simulink model "power_steppermotor"  (R2015b)
settings: Solver=FixedStepDiscrete  StartTime=0.0  StopTime=0.12  FixedStep=Ts  MaxStep=2e-6
PreLoadFcn:
  | assignin('base','Ts',0.5*1e-8);
InitFcn:
  | Ts=0.5*1e-8;
undefined symbols (not defined in the file): DiscIntNeverNeededParam, sigbuilder_block
libraries: powerlib x7
Description:
  | Copyright 2008-2015 The MathWorks, Inc.
settings Model: ExtModeAutoUpdateStatusClock=off  Creator=MathWorks  LastModifiedBy=YogurtSuee
settings DataIOCC: SaveFormat=Array  SignalLoggingSaveFormat=ModelDataLogs
settings OptimizationCC: ExpressionDepthLimit=2147483647  InitFltsAndDblsToZero=on
settings DebuggingCC: UnderspecifiedInitializationDetection=Classic  MergeDetectMultiDrivingBlocksExec=none  SignalResolutionControl=TryResolveAllWithWarning  SolverPrmCheckMsg=warning  FcnCallInpInsideContextMsg=UseLocalSettings  StateNameClashWarn=warning
settings HardwareCC: ProdBitPerPointer=32  ProdLargestAtomicFloat=None  ProdIntDivRoundTo=Undefined  ProdEndianess=Unspecified  ProdWordSize=32  ProdHWDeviceType=32-bit Generic
settings GRTTargetCC: GeneratePreprocessorConditionals=Disable all  CombineOutputUpdateFcns=off  GRTInterface=on
settings ConfigComp: CovModelRefEnable=Off  CovSFcnEnable=off

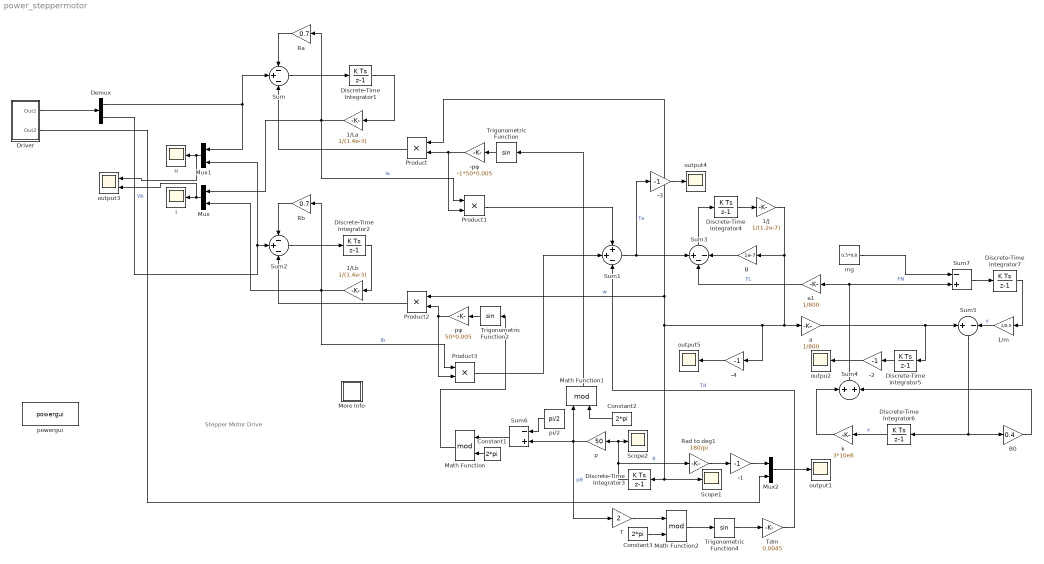
== system power_steppermotor ==
  note: Stepper Motor Drive
  -{1..4} (4 alike) : Gain  Gain=-1
  -pφ : Gain  Gain=-1*50*0.005
  1/J : Gain  Gain=1/(1.2e-7)
  1/La : Gain  Gain=1/(1.4e-3)
  1/Lb : Gain  Gain=1/(1.4e-3)
  1/m : Gain  Gain=1/0.5
  B : Gain  Gain=1e-7
  B0 : Gain  Gain=0.4
  Constant1 : Constant  Value=2*pi
  Constant2 : Constant  Value=2*pi
  Constant3 : Constant  Value=2*pi
  Demux : Demux  Outputs=2
  Discrete-Time Integrator{1..7} (7 alike) : DiscreteIntegrator  SampleTime=Ts  ICPrevOutput=DiscIntNeverNeededParam  ICPrevScaledInput=DiscIntNeverNeededParam
  Driver : Subsystem
  Math Function : Math  Operator=mod  SaturateOnIntegerOverflow=on
  Math Function1 : Math  Operator=mod  SaturateOnIntegerOverflow=on
  Math Function2 : Math  Operator=mod  SaturateOnIntegerOverflow=on
  More Info : Subsystem
      settings: OpenFcn=showdemo(bdroot(gcb))
      mask Display: disp('?')
  Mux : Mux  Inputs=2
  Mux1 : Mux  Inputs=2
  Mux2 : Mux  Inputs=2
  Product{,1..3} (4 alike) : Product
  Ra : Gain  Gain=0.7
  Rad to deg1 : Gain  Gain=180/pi
  Rb : Gain  Gain=0.7
  Scope1 : Scope
  Scope2 : Scope
  Sum : Sum  Inputs=-+-
  Sum1 : Sum  Inputs=++-
  Sum2 : Sum  Inputs=-+-
  Sum3 : Sum  Inputs=+--
  Sum4 : Sum
  Sum5 : Sum  Inputs=+-
  Sum6 : Sum  Inputs=-+
  Sum7 : Sum  Inputs=-+
  T : Gain  Gain=2
  Tdm : Gain  Gain=0.0045
  Trigonometric Function : Trigonometry
  Trigonometric Function2 : Trigonometry
  Trigonometric Function4 : Trigonometry
  a : Gain  Gain=1/800
  a1 : Gain  Gain=1/800
  i : Scope
  k : Gain  Gain=3*10e8
  mg : Constant  Value=0.5*9.8
  outpu2 : Scope
  output1 : Scope
  output3 : Scope  NumInputPorts=2
  output4 : Scope
  output5 : Scope
  p : Gain  Gain=50
  pi/2 : Constant  Value=pi/2
  powergui : powerlib/powergui  SimulationMode=Discrete  SolverType=Tustin/Backward Euler (TBE)  SampleTime=Ts  frequency=60  SPID=off  DisableSnubberDevices=off  DisableRonSwitches=off  DisableVfSwitches=off  SwTol=0  DisplayEquations=off  Interpol=off  ExternalGateDelay=off  methode=off  Ts=0  FunctionMessages=off  echomessages=off  HookPort=off  EnableUseOfTLC=off  x0status=blocks  frequencyindice=0  Pbase=100e6  ErrMax=1e-4  Iterations=50  UnitsV=V  UnitsW=W  buscounter=0  RestoreLinks=warning  ResistiveCurrentMeasurement=off  Frange=[0:2:500]  Ylog=off  Xlog=on  ShowGrid=off  save=off  variable=ZData  structure=0  ZoomFFT=on  StartTime=0.0  cycles=1  DisplayStyle=1  fundamental=60  FreqAxis=off  MaxFrequency=1000  frequencyindicesteady=1  RmsSteady=1  display=off
  pφ : Gain  Gain=50*0.005
  u : Scope
  wires:
  Discrete-Time Integrator1/1 -> 1/La/1
  Sum/1 -> Discrete-Time Integrator1/1
  Ra/1 -> Sum/1
  1/La/1 -> Product1/1, Mux/1, Ra/1  "Ia"
  Product/1 -> Sum/3
  -pφ/1 -> Product/2, Product1/2
  Product1/1 -> Sum1/1
  Discrete-Time Integrator2/1 -> 1/Lb/1
  Sum2/1 -> Discrete-Time Integrator2/1
  Rb/1 -> Sum2/1
  1/Lb/1 -> Product3/1, Mux/2, Rb/1  "Ib"
  Product2/1 -> Sum2/3
  pφ/1 -> Product2/2, Product3/2
  Product3/1 -> Sum1/2
  Tdm/1 -> Sum1/3  "Td"
  1/J/1 -> -4/1, Product2/1, Product/1, Discrete-Time Integrator3/1, Scope1/1, a/1, B/1  "w"
  Sum3/1 -> Discrete-Time Integrator4/1
  Discrete-Time Integrator4/1 -> 1/J/1
  Discrete-Time Integrator3/1 -> Rad to deg1/1, Scope2/1, p/1  "θ"
  p/1 -> Sum6/2, T/1, Math Function1/1  "pθ"
  pi/2/1 -> Sum6/1
  Mux/1 -> output3/2, i/1
  Mux1/1 -> output3/1, u/1
  Trigonometric Function4/1 -> Tdm/1
  Constant1/1 -> Math Function/2
  Sum6/1 -> Math Function/1
  Math Function/1 -> Trigonometric Function2/1
  Constant2/1 -> Math Function1/2
  Math Function1/1 -> Trigonometric Function/1
  Constant3/1 -> Math Function2/2
  T/1 -> Math Function2/1
  Math Function2/1 -> Trigonometric Function4/1
  Sum1/1 -> -3/1, Sum3/1  "Te"
  B/1 -> Sum3/3
  Trigonometric Function/1 -> -pφ/1
  Trigonometric Function2/1 -> pφ/1
  Demux/2 -> Mux1/2, Sum2/2  "Vb"
  Demux/1 -> Mux1/1, Sum/2
  Rad to deg1/1 -> -1/1
  Sum4/1 -> Sum7/2, a1/1  "FN"
  a/1 -> Discrete-Time Integrator5/1, Sum5/1
  mg/1 -> Sum7/1
  Sum7/1 -> Discrete-Time Integrator7/1
  Discrete-Time Integrator7/1 -> 1/m/1
  1/m/1 -> Sum5/2  "v"
  a1/1 -> Sum3/2  "TL"
  Sum5/1 -> Discrete-Time Integrator6/1, B0/1
  Discrete-Time Integrator6/1 -> k/1  "x"
  k/1 -> Sum4/1
  B0/1 -> Sum4/2
  Discrete-Time Integrator5/1 -> -2/1
  Driver/1(Out1) -> Demux/1
  Driver/2(Out2) -> Mux2/2
  Mux2/1 -> output1/1
  -1/1 -> Mux2/1
  -2/1 -> outpu2/1
  -3/1 -> output4/1
  -4/1 -> output5/1

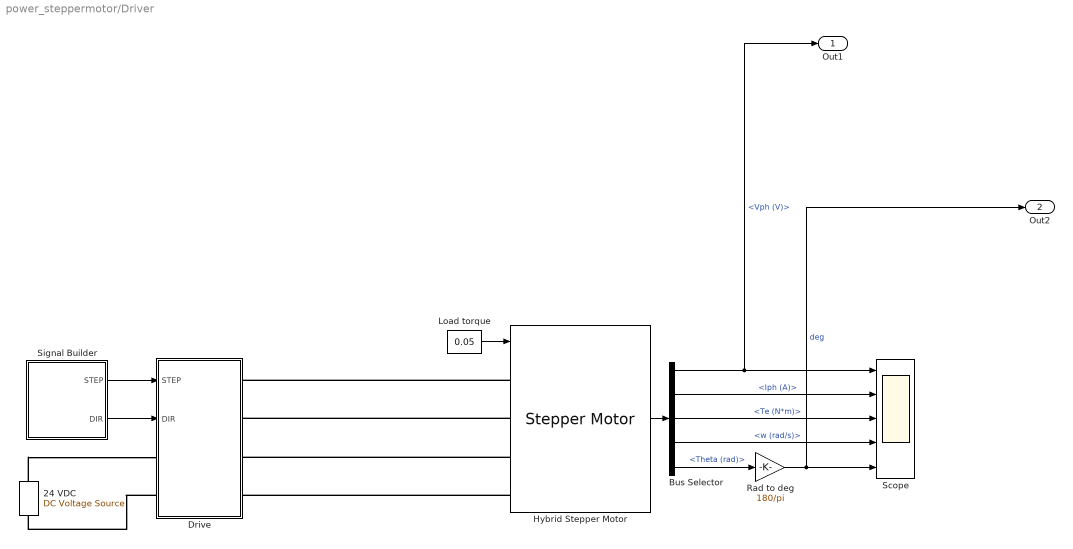
== system power_steppermotor/Driver ==
  24 VDC : powerlib/Electrical Sources/DC Voltage Source  Amplitude=24  Measurements=None
  Bus Selector : BusSelector  OutputSignals=Vph (V),Iph (A),Te (N*m),w (rad/s),Theta (rad)
  Drive : Subsystem  mask{Iref=2, step=200, Ts=Ts}
      mask prompts: Iref "Phase current (A)"; step "Stepping rate (step/s)"; Ts "Sampling time (s)"
      mask init:
      | Nstep=round(1/step/Ts);
  Hybrid Stepper Motor : powerlib/Machines/Stepper Motor  MotorType=Permanent-magnet / Hybrid  NumberOfPhases_1=2  NumberOfPhases_2=3  PresetModel_1=<empty>  PresetModel_2=<empty>  L=1.4e-3  Lmax=10e-3  Lmin=2e-3  R=0.7  Step_angle=1.8  Psim=0.005  Tdm=0.002  J=1.2e-7  B=1e-7*1000  w0=0  pos0=0  TsPowergui=0  TsBlock=-1
  Load torque : Constant  Value=0.05
  Rad to deg : Gain  Gain=180/pi
  Scope : Scope  NumInputPorts=5
  Signal Builder : Subsystem  Tag=STV Subsys  LoadFcn=sigbuilder_block('load');  StartFcn=sigbuilder_block('start');  StopFcn=sigbuilder_block('stop');  ClipboardFcn=sigbuilder_block('clipboard');  mask(Sigbuilder block){}
      mask help: Sigbuilder GUI
      mask init:
      | if ~strcmp(get_param(bdroot(gcbh),'SimulationStatus'),'stopped') tuvar = sigbuilder_block('maskInit'); end
      settings: CopyFcn=sigbuilder_block('copy');  DeleteFcn=sigbuilder_block('delete');  ModelCloseFcn=sigbuilder_block('modelClose');  PreSaveFcn=sigbuilder_block('preSave');  PauseFcn=sigbuilder_block('pause')  ContinueFcn=sigbuilder_block('continue')  NameChangeFcn=sigbuilder_block('namechange');  OpenFcn=sigbuilder_block('open',[162.75 86.25 550.5 363.75 ]);  CloseFcn=sigbuilder_block('close');
      mask Display: plot(0,0,100,100,[10,10,40,40,10],[80,20,20,80,80],[40,10],[50,50], [40,27,10],[65,72,56],[40,25,25,10],[28,28,43,43]);
  Out1 : Outport
  Out2 : Outport  Port=2
  wires:
  Signal Builder/1(STEP) -> Drive/1(STEP)
  Signal Builder/2(DIR) -> Drive/2(DIR)
  Hybrid Stepper Motor/1 -> Bus Selector/1
  Bus Selector/5 -> Rad to deg/1  "<Theta (rad)>"
  Bus Selector/4 -> Scope/4  "<w (rad/s)>"
  Bus Selector/3 -> Scope/3  "<Te (N*m)>"
  Bus Selector/2 -> Scope/2  "<Iph (A)>"
  Load torque/1 -> Hybrid Stepper Motor/1
  Bus Selector/1 -> Out1/1, Scope/1  "<Vph (V)>"
  Rad to deg/1 -> Out2/1, Scope/5  "deg"
  connections:
  24 VDC/RConn1 -- Drive/LConn1
  Hybrid Stepper Motor/LConn4 -- Drive/RConn4
  Hybrid Stepper Motor/LConn1 -- Drive/RConn1
  Drive/LConn2 -- 24 VDC/LConn1
  Hybrid Stepper Motor/LConn3 -- Drive/RConn3
  Hybrid Stepper Motor/LConn2 -- Drive/RConn2

== system power_steppermotor/More Info ==

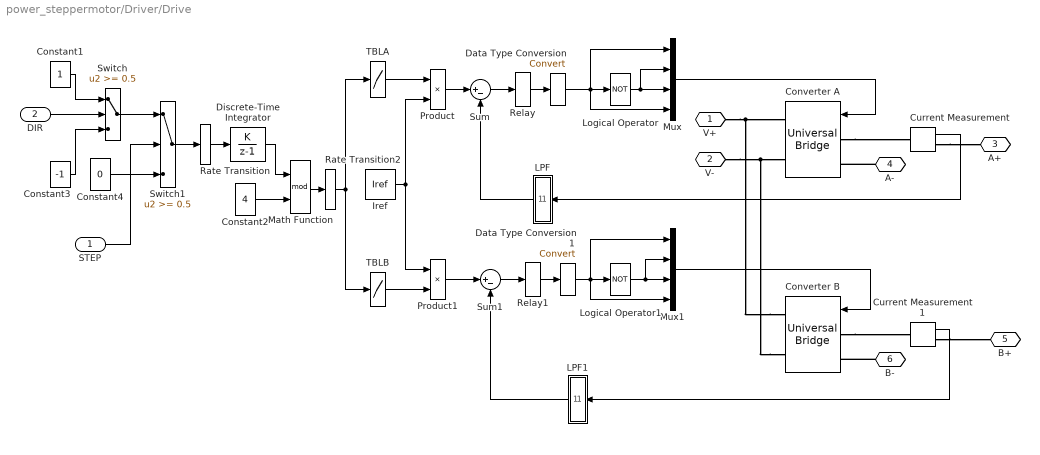
== system power_steppermotor/Driver/Drive ==
  STEP : Inport
  DIR : Inport  Port=2
  Constant1 : Constant  SampleTime=Ts
  Constant2 : Constant  Value=4  SampleTime=Nstep*Ts
  Constant3 : Constant  Value=-1  SampleTime=Ts
  Constant4 : Constant  Value=0  SampleTime=Ts
  Converter A : powerlib/Power Electronics/Universal Bridge  Arms=2  SnubberResistance=10000  SnubberCapacitance=inf  Device=MOSFET / Diodes  Ron=1e-3*10  Lon=0  ForwardVoltages="[  0  0  ]"  ForwardVoltage=0  GTOparameters=[ 10e-6 , 20e-6 ]  IGBTparameters=[ 0.5e-6 , 0.5e-6 ]  Measurements=None  Measurements_2=None  converterType=Rectifier
  Converter B : powerlib/Power Electronics/Universal Bridge  Arms=2  SnubberResistance=10000  SnubberCapacitance=inf  Device=MOSFET / Diodes  Ron=1e-3*10  Lon=0  ForwardVoltages="[  0  0  ]"  ForwardVoltage=0  GTOparameters=[ 10e-6 , 20e-6 ]  IGBTparameters=[ 0.5e-6 , 0.5e-6 ]  Measurements=None  Measurements_2=None  converterType=Rectifier
  Current Measurement : powerlib/Measurements/Current Measurement  PhasorSimulation=off  OutputType=Complex  PSBequivalent=0
  Current Measurement1 : powerlib/Measurements/Current Measurement  PhasorSimulation=off  OutputType=Complex  PSBequivalent=0
  Data Type Conversion : DataTypeConversion
  Data Type Conversion1 : DataTypeConversion
  Discrete-Time Integrator : DiscreteIntegrator  IntegratorMethod=Accumulation: Forward Euler  SampleTime=Nstep*Ts  ICPrevOutput=DiscIntNeverNeededParam  ICPrevScaledInput=DiscIntNeverNeededParam
  Iref : Constant  Value=Iref  SampleTime=Ts
  LPF : Subsystem  mask{fc=10000, Ts=Ts}
      mask prompts: fc "Cut-off frequency (Hz)"; Ts "Sampling time (s)"
      mask init:
      | % fa=tf(1,[1/2/pi/fc 1]);
      | % fn=c2d(fa,Ts);
      | % [NN,DD]=tfdata(fn,'v')
      | 
      | NN = [ 0,0.0609];
      | DD = [1.0000,-0.9391];
  LPF1 : Subsystem  mask{fc=10000, Ts=Ts}
      mask prompts: fc "Cut-off frequency (Hz)"; Ts "Sampling time (s)"
      mask init:
      | % fa=tf(1,[1/2/pi/fc 1]);
      | % fn=c2d(fa,Ts);
      | % [NN,DD]=tfdata(fn,'v')
      | 
      | NN = [ 0,0.0609];
      | DD = [1.0000,-0.9391];
  Logical Operator : Logic  Operator=NOT  AllPortsSameDT=off  OutDataTypeStr=boolean
  Logical Operator1 : Logic  Operator=NOT  AllPortsSameDT=off  OutDataTypeStr=boolean
  Math Function : Math  Operator=mod  SampleTime=Nstep*Ts  SaturateOnIntegerOverflow=on
  Mux : Mux
  Mux1 : Mux
  Product : Product  RndMeth=Zero
  Product1 : Product  RndMeth=Zero
  Rate Transition : RateTransition
  Rate Transition2 : RateTransition
  Relay : Relay  OnSwitchValue=0.01  OffSwitchValue=-0.01
  Relay1 : Relay  OnSwitchValue=0.01  OffSwitchValue=-0.01  OutDataTypeStr=Inherit: Inherit via back propagation
  Sum : Sum  Inputs=|+-  OutDataTypeStr=Inherit: Same as first input
  Sum1 : Sum  Inputs=|+-  OutDataTypeStr=Inherit: Same as first input
  Switch : Switch  Threshold=0.5  ZeroCross=off  SampleTime=Ts
  Switch1 : Switch  Threshold=0.5  ZeroCross=off  SampleTime=Ts
  TBLA : Lookup  InputValues=[0:3]  Table=[1 0 -1 0]  SampleTime=Ts
  TBLB : Lookup  InputValues=[0:3]  Table=[0 1 0 -1]  SampleTime=Ts
  V+ : PMIOPort  Port=1  Side=Left
  V- : PMIOPort  Port=2  Side=Left
  A+ : PMIOPort  Port=3  Side=Right
  A- : PMIOPort  Port=4  Side=Right
  B+ : PMIOPort  Port=5  Side=Right
  B- : PMIOPort  Port=6  Side=Right
  wires:
  Constant4/1 -> Switch1/3
  Switch1/1 -> Rate Transition/1
  Switch/1 -> Switch1/1
  STEP/1 -> Switch1/2
  DIR/1 -> Switch/2
  Rate Transition2/1 -> TBLB/1, TBLA/1
  Math Function/1 -> Rate Transition2/1
  Product1/1 -> Sum1/1
  Product/1 -> Sum/1
  Rate Transition/1 -> Discrete-Time Integrator/1
  Constant3/1 -> Switch/3
  Constant1/1 -> Switch/1
  Discrete-Time Integrator/1 -> Math Function/1
  Constant2/1 -> Math Function/2
  Iref/1 -> Product1/1, Product/2
  TBLB/1 -> Product1/2
  TBLA/1 -> Product/1
  LPF1/1(O) -> Sum1/2
  LPF/1(O) -> Sum/2
  Data Type Conversion1/1 -> Mux1/4, Mux1/1, Logical Operator1/1
  Data Type Conversion/1 -> Logical Operator/1, Mux/4, Mux/1
  Current Measurement1/1 -> LPF1/1(I)
  Sum1/1 -> Relay1/1
  Mux1/1 -> Converter B/1
  Logical Operator1/1 -> Mux1/2, Mux1/3
  Relay1/1 -> Data Type Conversion1/1
  Mux/1 -> Converter A/1
  Logical Operator/1 -> Mux/2, Mux/3
  Relay/1 -> Data Type Conversion/1
  Current Measurement/1 -> LPF/1(I)
  Sum/1 -> Relay/1
  connections:
  Converter B/RConn2 -- Converter A/RConn2 -- V-/RConn1
  Converter B/RConn1 -- Converter A/RConn1 -- V+/RConn1
  Current Measurement1/RConn1 -- B+/RConn1
  Converter B/LConn1 -- Current Measurement1/LConn1
  Current Measurement/RConn1 -- A+/RConn1
  Converter A/LConn1 -- Current Measurement/LConn1
  B-/RConn1 -- Converter B/LConn2
  A-/RConn1 -- Converter A/LConn2

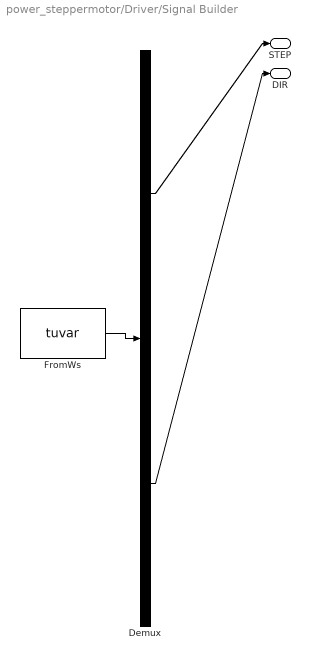
== system power_steppermotor/Driver/Signal Builder ==
  Demux : Demux  Tag=STV Demux  Outputs=2
  FromWs : FromWorkspace  Tag=STV FromWs  VariableName=tuvar  SampleTime=0
      SigBuilderData=|
      | common.afterFinalStr = 'Extrapolate'
      | common.sampleTime = 0
      | dataSet.timeRange = [0 4]
      | dataSet.name = 'Group 1'
      | sbobj.Groups.Name = 'Group 1'
      | sbobj.Groups.Signals(1).Name = 'STEP'
      | sbobj.Groups.Signals(1).XData = [0 0.08 0.08 4]
      | sbobj.Groups.Signals(1).YData = [1 1 0 0]
      | sbobj.Groups.Signals(2).Name = 'DIR'
      | sbobj.Groups.Signals(2).XData = [0 0.04 0.04 4]
      | sbobj.Groups.Signals(2).YData = [1 1 0 0]
      | sbobj.Groups.TimeRange = [0 4]
  STEP : Outport  Tag=STV Outport
  DIR : Outport  Tag=STV Outport  Port=2
  wires:
  FromWs/1 -> Demux/1
  Demux/1 -> STEP/1
  Demux/2 -> DIR/1

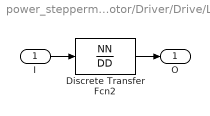
== system power_steppermotor/Driver/Drive/LPF ==
  I : Inport
  Discrete Transfer Fcn2 : DiscreteTransferFcn  Numerator=NN  Denominator=DD  SampleTime=Ts
  O : Outport
  wires:
  Discrete Transfer Fcn2/1 -> O/1
  I/1 -> Discrete Transfer Fcn2/1

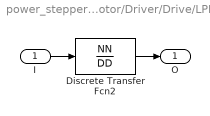
== system power_steppermotor/Driver/Drive/LPF1 ==
  I : Inport
  Discrete Transfer Fcn2 : DiscreteTransferFcn  Numerator=NN  Denominator=DD  SampleTime=Ts
  O : Outport
  wires:
  I/1 -> Discrete Transfer Fcn2/1
  Discrete Transfer Fcn2/1 -> O/1
